simulink model "bonnuoc_fuzzy_sim"  (R2019a)
settings: Solver=ode3  StartTime=0.0  StopTime=50  FixedStep=0.01  RelTol=1e-3
libraries: fuzblock x1
settings Model: Creator=ASUS  LastModifiedBy=ASUS
settings DataIOCC: ReturnWorkspaceOutputs=off

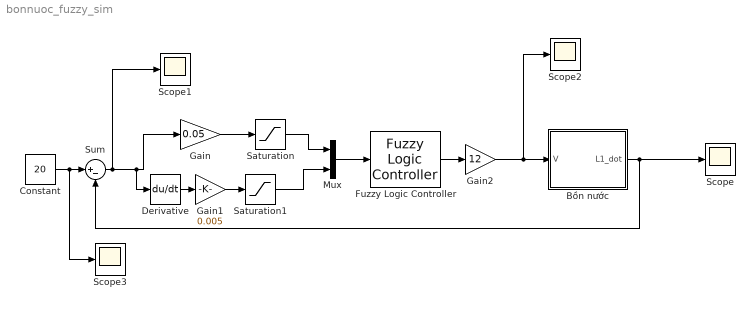
== system bonnuoc_fuzzy_sim ==
  Bồn nước : Subsystem
  Constant : Constant  Value=20
  Derivative : Derivative
  Fuzzy Logic Controller : fuzblock/Fuzzy Logic  Controller  FIS='fuzzy_of_tamcute.fis'  OutputSampleNumber=101  DataType=double  FuzzifiedInputs=off  RuleFiringStrengths=off  RuleOutputs=off  AggregatedOutputs=off  SimulateUsing=Interpreted execution  OutOfRangeInputValueMessage=warning  NoRuleFiredMessage=warning  EmptyOutputFuzzySetMessage=warning
  Gain : Gain  Gain=0.05
  Gain1 : Gain  Gain=0.005
  Gain2 : Gain  Gain=12
  Mux : Mux  Inputs=2
  Saturation : Saturate  UpperLimit=1  LowerLimit=-1
  Saturation1 : Saturate  UpperLimit=1  LowerLimit=-1
  Scope{,1..3} (4 alike) : Scope
  Sum : Sum  Inputs=|+-
  wires:
  Mux/1 -> Fuzzy Logic Controller/1
  Fuzzy Logic Controller/1 -> Gain2/1
  Gain2/1 -> Scope2/1, Bồn nước/1(V)
  Gain/1 -> Saturation/1
  Saturation/1 -> Mux/1
  Saturation1/1 -> Mux/2
  Gain1/1 -> Saturation1/1
  Bồn nước/1(L1_dot) -> Scope/1, Sum/2
  Sum/1 -> Derivative/1, Gain/1, Scope1/1
  Constant/1 -> Scope3/1, Sum/1
  Derivative/1 -> Gain1/1

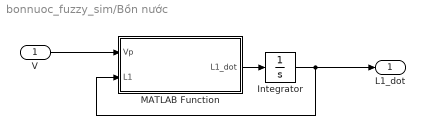
== system bonnuoc_fuzzy_sim/Bồn nước ==
  V : Inport
  Integrator : Integrator
  MATLAB Function : MATLAB Function  TreatAsAtomicUnit=on
  L1_dot : Outport
  wires:
  MATLAB Function/1(L1_dot) -> Integrator/1
  V/1 -> MATLAB Function/1(Vp)
  Integrator/1 -> L1_dot/1, MATLAB Function/2(L1)

== matlab function bonnuoc_fuzzy_sim/Bồn nước/MATLAB Function ==
  data: Vp input; L1 input; L1_dot output
function L1_dot= BON_NUOC(Vp,L1)
Km=4.6;
A1=15.5179;
a1=0.2;
g=9.8;
%equation
L1_dot=-(a1/A1)*sqrt(2*g*L1)+(Km/A1)*Vp;
